simulink model "feedback_lin_RLS_soloR"  (R2023b)
settings: Solver=VariableStepAuto  StartTime=0.0  StopTime=10  RelTol=1e-3
undefined symbols (not defined in the file): A_ob, B_ob, C_ob, D_ob, k_aero, k_mag, k_mag_mod, Lc, Lc_mod, m, Rtot, Rtot_mod, theta, x1_eq0, x2_eq0, y0
libraries: simulink x6
settings Model: Creator=lollo  LastModifiedBy=lollo

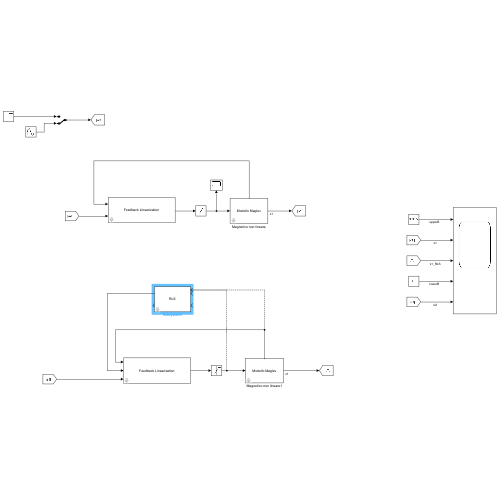
[thumbnail: Simulink's stored preview of the top-level diagram]
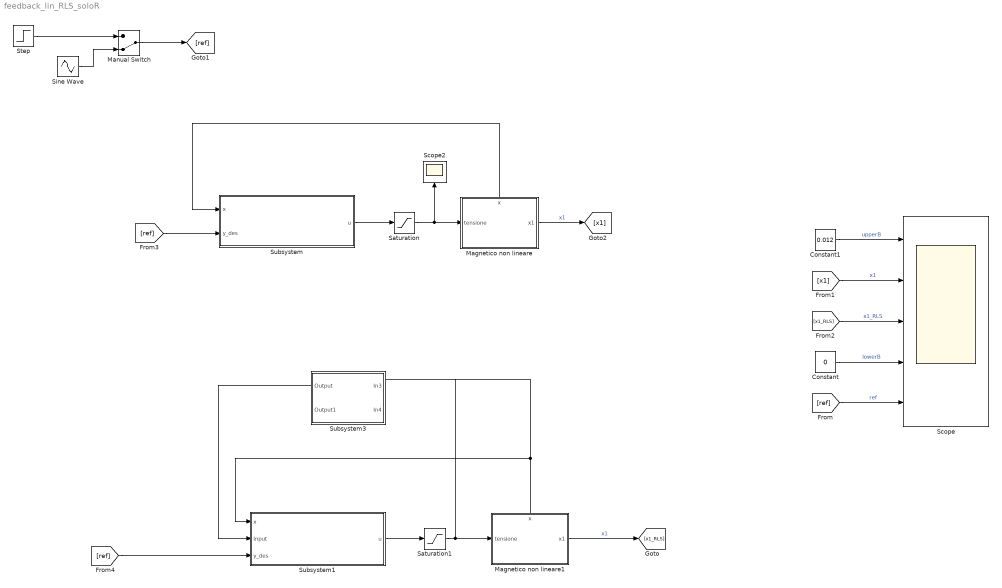
== system feedback_lin_RLS_soloR ==
  Constant : Constant  Value=0
  Constant1 : Constant  Value=0.012
  Magnetico non lineare : Subsystem  mask{dist=off, obs=on}
      mask prompts: dist "Aggiungere Disturbi"; obs "Observer invece di misura"
      settings: PortSchema="{\"entries\":[{\"content\":{\"sides\":[{\"content\":{\"connectorIds\":[\"In1\"]},\"type\":\"ConnectorPlacement.EquallySpacedRectSide\",\"uuid\":\"4c2628b7-19c4-4753-accd-078547eff280\"},{\"content\":{\"connectorIds\":[\"Out1\"],\"side\":\"RIGHT\"},\"type\":\"ConnectorPlacement.EquallySpacedRectSide\",\"uuid\":\"46f8a782-99b4-4db5-ac9e-879226864e1a\"},{\"content\":{\"connectorIds\":[\"Out2\"],\"side\":\"TOP\"},\"type\":\"ConnectorPlacement.EquallySpacedRectSide\",\"uuid\":\"e9ea6a3a-0b10-4f27-be26-5b91ce6de957\"}]},\"type\":\"ConnectorPlacement.EquallySpacedConnector\",\"uuid\":\"8380a659-82e1-48e4-be7e-4b84feeb9f50\"}],\"packageUris\":[\"http://schema.mathworks.com/mf0/Connector/R2020b\"],\"version\":\"1.0\"}"
      mask DialogControl DescGroupVar Prompt: MAGLEV
      mask DialogControl Maglev Prompt: Possibilità di aggiungere disturbi alla misura o di considerare gli observer (solo ridotto alla velocità). Inoltre possibilità di modificare i parametri del modello per testare robustezza
      mask DialogControl Disturbi Prompt: Disturbi
      mask Display: disp('Modello Maglev')
  Magnetico non lineare1 : Subsystem  mask{dist=on, obs=on}
      mask prompts: dist "Aggiungere Disturbi"; obs "Observer invece di misura"
      settings: PortSchema="{\"entries\":[{\"content\":{\"sides\":[{\"content\":{\"connectorIds\":[\"In1\"]},\"type\":\"ConnectorPlacement.EquallySpacedRectSide\",\"uuid\":\"4c2628b7-19c4-4753-accd-078547eff280\"},{\"content\":{\"connectorIds\":[\"Out1\"],\"side\":\"RIGHT\"},\"type\":\"ConnectorPlacement.EquallySpacedRectSide\",\"uuid\":\"46f8a782-99b4-4db5-ac9e-879226864e1a\"},{\"content\":{\"connectorIds\":[\"Out2\"],\"side\":\"TOP\"},\"type\":\"ConnectorPlacement.EquallySpacedRectSide\",\"uuid\":\"e9ea6a3a-0b10-4f27-be26-5b91ce6de957\"}]},\"type\":\"ConnectorPlacement.EquallySpacedConnector\",\"uuid\":\"8380a659-82e1-48e4-be7e-4b84feeb9f50\"}],\"packageUris\":[\"http://schema.mathworks.com/mf0/Connector/R2020b\"],\"version\":\"1.0\"}"
      mask DialogControl DescGroupVar Prompt: MAGLEV
      mask DialogControl Maglev Prompt: Possibilità di aggiungere disturbi alla misura o di considerare gli observer (solo ridotto alla velocità). Inoltre possibilità di modificare i parametri del modello per testare robustezza
      mask DialogControl Disturbi Prompt: Disturbi
      mask Display: disp('Modello Maglev')
  Manual Switch : ManualSwitch  CurrentSetting=0
  Saturation : Saturate  UpperLimit=23  LowerLimit=0
  Saturation1 : Saturate  UpperLimit=23  LowerLimit=0
  Scope : Scope  NumInputPorts=5
  Scope2 : Scope
  Sine Wave : Sin  Amplitude=0.001  Bias=0.003  Frequency=10  SampleTime=0
  Step : Step  Time=0  After=0.003  SampleTime=0
  Subsystem : Subsystem  mask{tau=0.003, p1=-100, p2=-60, p3=-70}
      mask DialogControl DescGroupVar Prompt: Feedback Linearization
      mask DialogControl DescTextVar Prompt: Tau corrisponde al tempo caratteristico del filtro per il calcolo delle derivate. k1, k2, k3 sono i poli della feedback linearization dei rispettivi stati
      mask Display: disp('Feedback Linearization')
  Subsystem1 : Subsystem  mask{tau=0.003, p1=-40, p2=-50, p3=-50}
      mask DialogControl DescGroupVar Prompt: Feedback Linearization
      mask DialogControl DescTextVar Prompt: Tau corrisponde al tempo caratteristico del filtro per il calcolo delle derivate. k1, k2, k3 sono i poli della feedback linearization dei rispettivi stati
      mask Display: disp('Feedback Linearization')
  Subsystem3 : Subsystem
      mask Display: disp('RLS')
  wires:
  Magnetico non lineare/2(x) -> Subsystem/1(x)
  Manual Switch/1 -> [ref]
  Subsystem/1(u) -> Saturation/1
  Saturation/1 -> Magnetico non lineare/1(tensione), Scope2/1
  Step/1 -> Manual Switch/1
  Sine Wave/1 -> Manual Switch/2
  Saturation1/1 -> Magnetico non lineare1/1(tensione)
  Magnetico non lineare1/2(x) -> Subsystem1/1(x)
  [ref] -> Subsystem1/3(y_des)
  Subsystem3/1(Output) -> Subsystem1/2(Input)
  Constant/1 -> Scope/4  "lowerB"
  [x1] -> Scope/2  "x1"
  [ref] -> Scope/5  "ref"
  Constant1/1 -> Scope/1  "upperB"
  Magnetico non lineare/1(x1) -> [x1]  "x1"
  [x1_RLS] -> Scope/3  "x1_RLS"
  Magnetico non lineare1/1(x1) -> [x1_RLS]  "x1"
  [ref] -> Subsystem/2(y_des)
  Subsystem1/1(u) -> Saturation1/1

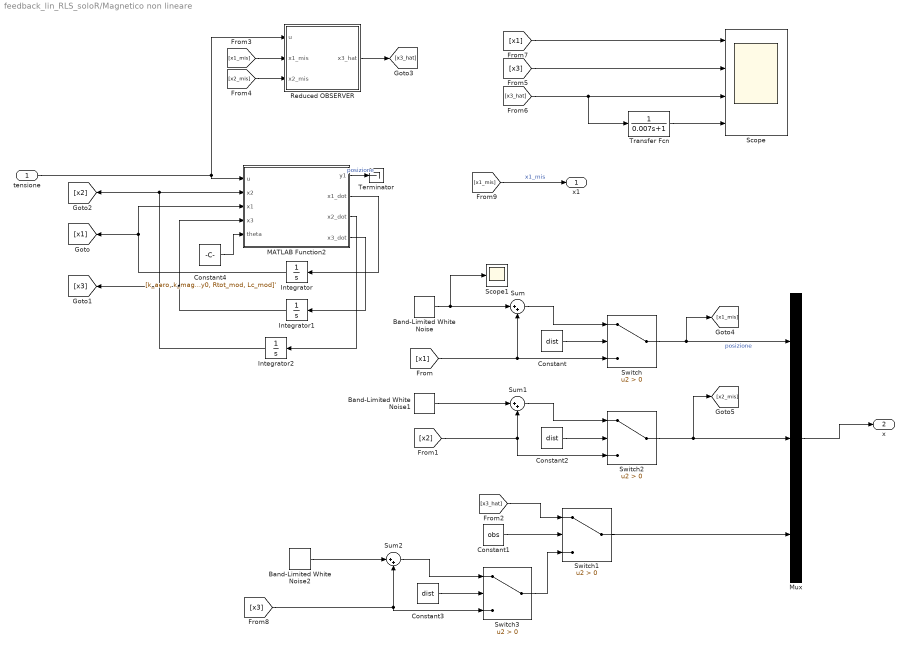
== system feedback_lin_RLS_soloR/Magnetico non lineare ==
  tensione : Inport
  Band-Limited White Noise : simulink/Sources/Band-Limited White Noise  Cov=[1e-10*0.002]  Ts=0.002  seed=[23341]
  Band-Limited White Noise1 : simulink/Sources/Band-Limited White Noise  Cov=[8.9934e-11*0.002]  Ts=0.002  seed=[23341]
  Band-Limited White Noise2 : simulink/Sources/Band-Limited White Noise  Cov=[8.9934e-11*0.002]  Ts=0.002  seed=[23341]
  Constant : Constant  Value=dist
  Constant1 : Constant  Value=obs
  Constant2 : Constant  Value=dist
  Constant3 : Constant  Value=dist
  Constant4 : Constant  Value=[k_aero, k_mag_mod, m, y0, Rtot_mod, Lc_mod]'
  Integrator : Integrator
  Integrator1 : Integrator
  Integrator2 : Integrator
  MATLAB Function2 : MATLAB Function  TreatAsAtomicUnit=on
  Mux : Mux  Inputs=3
  Reduced OBSERVER : Subsystem
  Scope : Scope  NumInputPorts=4
  Scope1 : Scope
  Sum : Sum  Inputs=|++
  Sum1 : Sum  Inputs=|++
  Sum2 : Sum  Inputs=|++
  Switch{,1..3} (4 alike) : Switch  Criteria=u2 > Threshold  SaturateOnIntegerOverflow=off  InputSameDT=off
  Terminator : Terminator
  Transfer Fcn : TransferFcn  Denominator=[0.007 1]
  x1 : Outport
  x : Outport  Port=2
  wires:
  tensione/1 -> Reduced OBSERVER/1(u), MATLAB Function2/1(u)
  Switch/1 -> [x1_mis], Mux/1  "posizione"
  MATLAB Function2/2(x1_dot) -> Integrator/1
  Integrator/1 -> MATLAB Function2/3(x1), [x1]
  MATLAB Function2/4(x3_dot) -> Integrator1/1
  Integrator1/1 -> [x3], MATLAB Function2/4(x3)
  [x1] -> Sum/2, Switch/3
  [x3_hat] -> Switch1/1
  Mux/1 -> x/1
  MATLAB Function2/3(x2_dot) -> Integrator2/1
  [x1_mis] -> Reduced OBSERVER/2(x1_mis)
  [x2_mis] -> Reduced OBSERVER/3(x2_mis)
  Reduced OBSERVER/1(x3_hat) -> [x3_hat]
  [x3_hat] -> Transfer Fcn/1, Scope/3
  [x3] -> Scope/2
  Integrator2/1 -> [x2], MATLAB Function2/2(x2)
  [x1] -> Scope/1
  Constant/1 -> Switch/2
  Band-Limited White Noise/1 -> Scope1/1, Sum/1
  Sum/1 -> Switch/1
  Constant1/1 -> Switch1/2
  Switch1/1 -> Mux/3
  Constant2/1 -> Switch2/2
  Switch2/1 -> [x2_mis], Mux/2
  Band-Limited White Noise1/1 -> Sum1/1
  Sum1/1 -> Switch2/1
  [x2] -> Sum1/2, Switch2/3
  Constant3/1 -> Switch3/2
  Switch3/1 -> Switch1/3
  Band-Limited White Noise2/1 -> Sum2/1
  Sum2/1 -> Switch3/1
  [x3] -> Sum2/2, Switch3/3
  Constant4/1 -> MATLAB Function2/5(theta)
  Transfer Fcn/1 -> Scope/4
  [x1_mis] -> x1/1  "x1_mis"
  MATLAB Function2/1(y1) -> Terminator/1  "posizione"

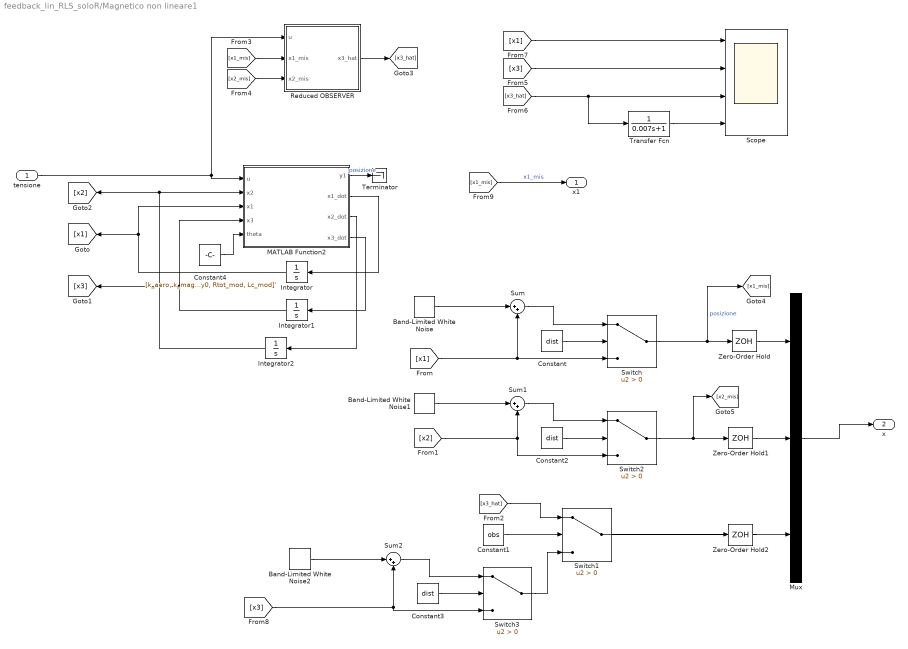
== system feedback_lin_RLS_soloR/Magnetico non lineare1 ==
  tensione : Inport
  Band-Limited White Noise : simulink/Sources/Band-Limited White Noise  Cov=[1e-8*0.002]  Ts=0.002  seed=[23341]
  Band-Limited White Noise1 : simulink/Sources/Band-Limited White Noise  Cov=[8.9934e-11*0.002]  Ts=0.002  seed=[23341]
  Band-Limited White Noise2 : simulink/Sources/Band-Limited White Noise  Cov=[8.9934e-11*0.002]  Ts=0.002  seed=[23341]
  Constant : Constant  Value=dist
  Constant1 : Constant  Value=obs
  Constant2 : Constant  Value=dist
  Constant3 : Constant  Value=dist
  Constant4 : Constant  Value=[k_aero, k_mag_mod, m, y0, Rtot_mod, Lc_mod]'
  Integrator : Integrator
  Integrator1 : Integrator
  Integrator2 : Integrator
  MATLAB Function2 : MATLAB Function  TreatAsAtomicUnit=on
  Mux : Mux  Inputs=3
  Reduced OBSERVER : Subsystem
  Scope : Scope  NumInputPorts=4
  Sum : Sum  Inputs=|++
  Sum1 : Sum  Inputs=|++
  Sum2 : Sum  Inputs=|++
  Switch{,1..3} (4 alike) : Switch  Criteria=u2 > Threshold  SaturateOnIntegerOverflow=off  InputSameDT=off
  Terminator : Terminator
  Transfer Fcn : TransferFcn  Denominator=[0.007 1]
  Zero-Order Hold : ZeroOrderHold  SampleTime=0.002
  Zero-Order Hold1 : ZeroOrderHold  SampleTime=0.002
  Zero-Order Hold2 : ZeroOrderHold  SampleTime=0.002
  x1 : Outport
  x : Outport  Port=2
  wires:
  tensione/1 -> Reduced OBSERVER/1(u), MATLAB Function2/1(u)
  Switch/1 -> [x1_mis], Zero-Order Hold/1  "posizione"
  MATLAB Function2/2(x1_dot) -> Integrator/1
  Integrator/1 -> MATLAB Function2/3(x1), [x1]
  MATLAB Function2/4(x3_dot) -> Integrator1/1
  Integrator1/1 -> [x3], MATLAB Function2/4(x3)
  [x1] -> Sum/2, Switch/3
  [x3_hat] -> Switch1/1
  Mux/1 -> x/1
  MATLAB Function2/3(x2_dot) -> Integrator2/1
  [x1_mis] -> Reduced OBSERVER/2(x1_mis)
  [x2_mis] -> Reduced OBSERVER/3(x2_mis)
  Reduced OBSERVER/1(x3_hat) -> [x3_hat]
  [x3_hat] -> Transfer Fcn/1, Scope/3
  [x3] -> Scope/2
  Integrator2/1 -> [x2], MATLAB Function2/2(x2)
  [x1] -> Scope/1
  Constant/1 -> Switch/2
  Band-Limited White Noise/1 -> Sum/1
  Sum/1 -> Switch/1
  Constant1/1 -> Switch1/2
  Switch1/1 -> Zero-Order Hold2/1
  Constant2/1 -> Switch2/2
  Switch2/1 -> [x2_mis], Zero-Order Hold1/1
  Band-Limited White Noise1/1 -> Sum1/1
  Sum1/1 -> Switch2/1
  [x2] -> Sum1/2, Switch2/3
  Constant3/1 -> Switch3/2
  Switch3/1 -> Switch1/3
  Band-Limited White Noise2/1 -> Sum2/1
  Sum2/1 -> Switch3/1
  [x3] -> Sum2/2, Switch3/3
  Constant4/1 -> MATLAB Function2/5(theta)
  Transfer Fcn/1 -> Scope/4
  [x1_mis] -> x1/1  "x1_mis"
  MATLAB Function2/1(y1) -> Terminator/1  "posizione"
  Zero-Order Hold/1 -> Mux/1
  Zero-Order Hold1/1 -> Mux/2
  Zero-Order Hold2/1 -> Mux/3

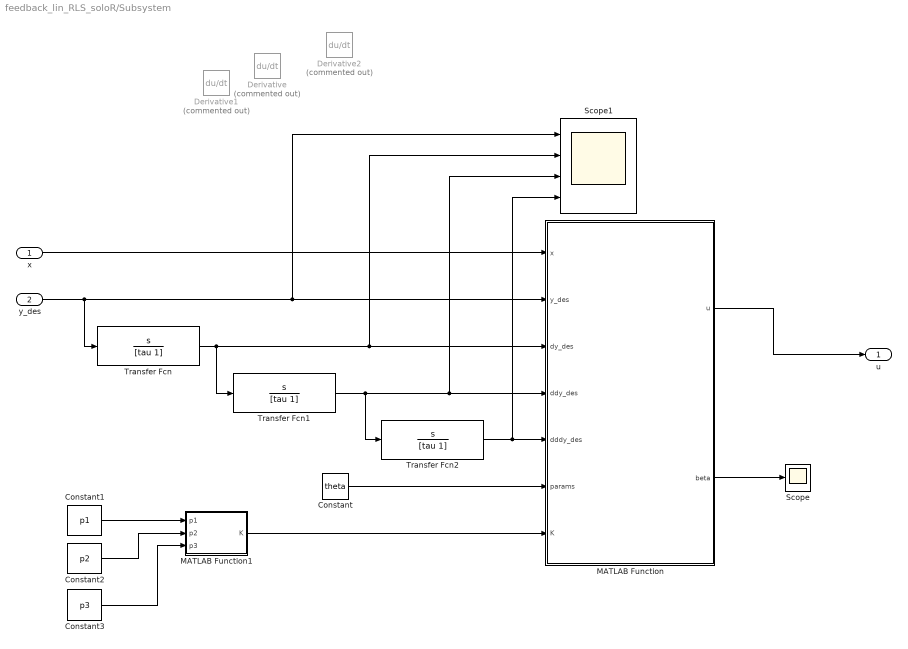
== system feedback_lin_RLS_soloR/Subsystem ==
  x : Inport
  y_des : Inport  Port=2
  Constant : Constant  Value=theta
  Constant1 : Constant  Value=p1
  Constant2 : Constant  Value=p2
  Constant3 : Constant  Value=p3
  Derivative : Derivative  Commented=on
  Derivative1 : Derivative  Commented=on
  Derivative2 : Derivative  Commented=on
  MATLAB Function : MATLAB Function  TreatAsAtomicUnit=on
  MATLAB Function1 : MATLAB Function  TreatAsAtomicUnit=on
  Scope : Scope
  Scope1 : Scope  NumInputPorts=4
  Transfer Fcn : TransferFcn  Numerator=[1 0]  Denominator=[tau 1]
  Transfer Fcn1 : TransferFcn  Numerator=[1 0]  Denominator=[tau 1]
  Transfer Fcn2 : TransferFcn  Numerator=[1 0]  Denominator=[tau 1]
  u : Outport
  wires:
  y_des/1 -> Transfer Fcn/1, MATLAB Function/2(y_des), Scope1/1
  x/1 -> MATLAB Function/1(x)
  MATLAB Function/1(u) -> u/1
  Transfer Fcn/1 -> MATLAB Function/3(dy_des), Scope1/2, Transfer Fcn1/1
  Constant/1 -> MATLAB Function/6(params)
  Transfer Fcn1/1 -> Transfer Fcn2/1, Scope1/3, MATLAB Function/4(ddy_des)
  MATLAB Function/2(beta) -> Scope/1
  Transfer Fcn2/1 -> Scope1/4, MATLAB Function/5(dddy_des)
  MATLAB Function1/1(K) -> MATLAB Function/7(K)
  Constant3/1 -> MATLAB Function1/3(p3)
  Constant2/1 -> MATLAB Function1/2(p2)
  Constant1/1 -> MATLAB Function1/1(p1)

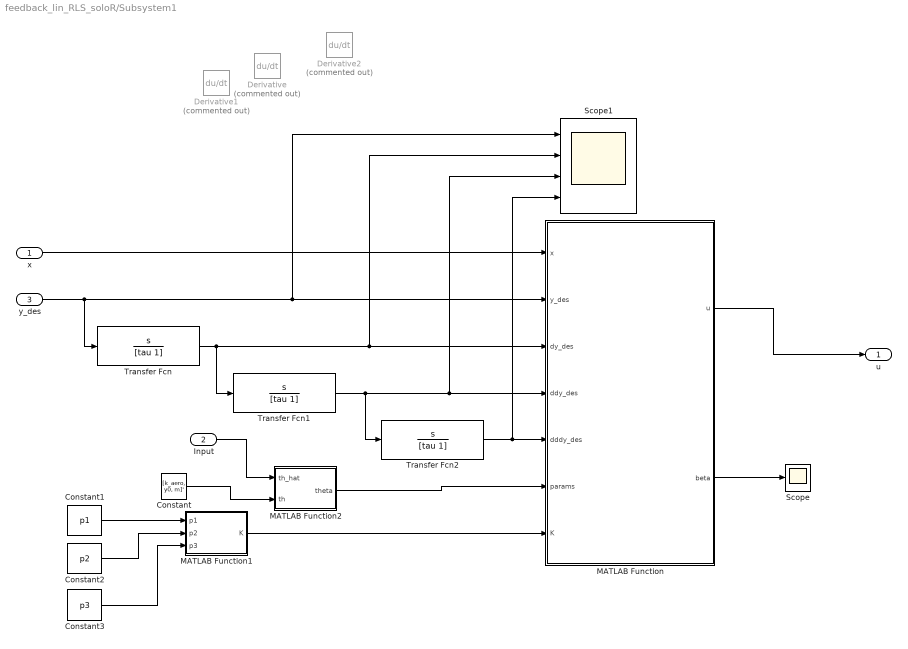
== system feedback_lin_RLS_soloR/Subsystem1 ==
  x : Inport
  Input : Inport  Port=2
  y_des : Inport  Port=3
  Constant : Constant  Value=[k_aero, y0, m]'
  Constant1 : Constant  Value=p1
  Constant2 : Constant  Value=p2
  Constant3 : Constant  Value=p3
  Derivative : Derivative  Commented=on
  Derivative1 : Derivative  Commented=on
  Derivative2 : Derivative  Commented=on
  MATLAB Function : MATLAB Function  TreatAsAtomicUnit=on
  MATLAB Function1 : MATLAB Function  TreatAsAtomicUnit=on
  MATLAB Function2 : MATLAB Function  TreatAsAtomicUnit=on
  Scope : Scope
  Scope1 : Scope  NumInputPorts=4
  Transfer Fcn : TransferFcn  Numerator=[1 0]  Denominator=[tau 1]
  Transfer Fcn1 : TransferFcn  Numerator=[1 0]  Denominator=[tau 1]
  Transfer Fcn2 : TransferFcn  Numerator=[1 0]  Denominator=[tau 1]
  u : Outport
  wires:
  y_des/1 -> Transfer Fcn/1, MATLAB Function/2(y_des), Scope1/1
  x/1 -> MATLAB Function/1(x)
  MATLAB Function/1(u) -> u/1
  Transfer Fcn/1 -> MATLAB Function/3(dy_des), Scope1/2, Transfer Fcn1/1
  MATLAB Function2/1(theta) -> MATLAB Function/6(params)
  Transfer Fcn1/1 -> Transfer Fcn2/1, Scope1/3, MATLAB Function/4(ddy_des)
  MATLAB Function/2(beta) -> Scope/1
  Transfer Fcn2/1 -> Scope1/4, MATLAB Function/5(dddy_des)
  MATLAB Function1/1(K) -> MATLAB Function/7(K)
  Constant3/1 -> MATLAB Function1/3(p3)
  Constant2/1 -> MATLAB Function1/2(p2)
  Constant1/1 -> MATLAB Function1/1(p1)
  Input/1 -> MATLAB Function2/1(th_hat)
  Constant/1 -> MATLAB Function2/2(th)

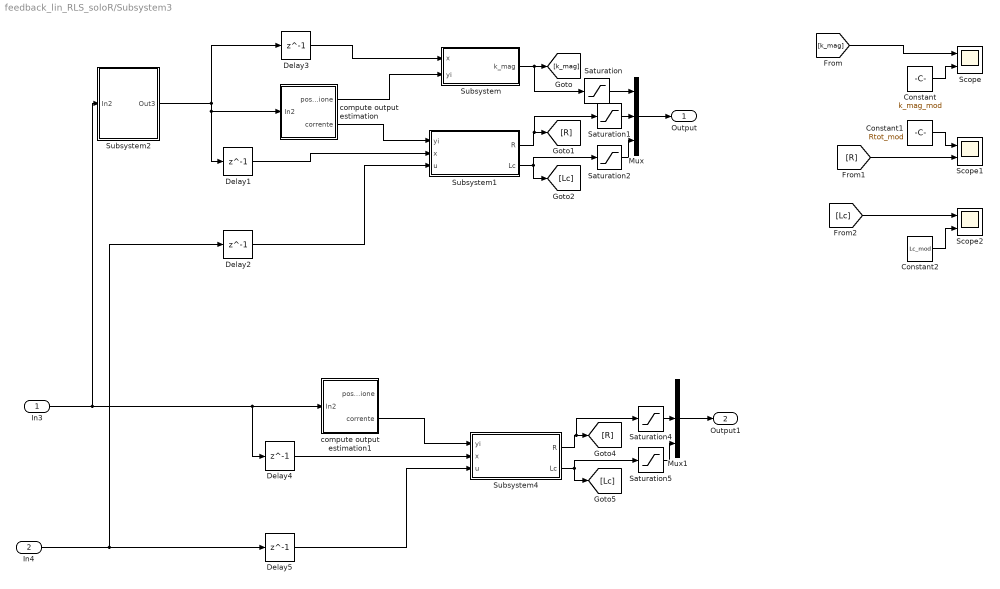
== system feedback_lin_RLS_soloR/Subsystem3 ==
  In3 : Inport
  In4 : Inport  Port=2
  Constant : Constant  Value=k_mag_mod
  Constant1 : Constant  Value=Rtot_mod
  Constant2 : Constant  Value=Lc_mod
  Delay{1..2,4..5} (4 alike) : Delay  DelayLength=1  InitialCondition=0
  Delay3 : Delay  DelayLength=1  InitialCondition=[0, 0, 0]'
  Mux : Mux  Inputs=3
  Mux1 : Mux  Inputs=3
  Saturation : Saturate  UpperLimit=1e-4  LowerLimit=1e-6
  Saturation1 : Saturate  UpperLimit=20  LowerLimit=0
  Saturation2 : Saturate  UpperLimit=2  LowerLimit=0
  Saturation4 : Saturate  UpperLimit=20  LowerLimit=0
  Saturation5 : Saturate  UpperLimit=2  LowerLimit=0
  Scope : Scope  NumInputPorts=2
  Scope1 : Scope  NumInputPorts=2
  Scope2 : Scope  NumInputPorts=2
  Subsystem : Subsystem  mask{th0=k_mag, S0=eye(1)/100, mu=0.98}
      mask prompts: th0 "Theta init"; mu "Forgetting factor"
      mask Display: disp('RLS (k_mag)')
  Subsystem1 : Subsystem  mask{th0=[Rtot; Lc], S0=eye(2)/10, mu=0.99}
      mask prompts: th0 "Theta init"; mu "Forgetting Factor"
      mask Display: disp('RLS (R, Lc)')
  Subsystem2 : Subsystem
  Subsystem4 : Subsystem  mask{th0=[Rtot; Lc], S0=eye(2)/10, mu=0.99}
      mask prompts: th0 "Theta init"; mu "Forgetting Factor"
      mask Display: disp('RLS (R, Lc)')
  compute output estimation : Subsystem
  compute output estimation1 : Subsystem
  Output : Outport
  Output1 : Outport  Port=2
  wires:
  Delay2/1 -> Subsystem1/3(u)
  Delay3/1 -> Subsystem/1(x)
  compute output estimation/1(posizione) -> Subsystem/2(yi)
  compute output estimation/2(corrente) -> Subsystem1/1(yi)
  Delay1/1 -> Subsystem1/2(x)
  Constant/1 -> Scope/2
  Constant1/1 -> Scope1/1
  Constant2/1 -> Scope2/2
  Subsystem/1(k_mag) -> Saturation/1, [k_mag]
  Subsystem1/1(R) -> Saturation1/1, [R]
  Subsystem1/2(Lc) -> [Lc], Saturation2/1
  [k_mag] -> Scope/1
  [R] -> Scope1/2
  [Lc] -> Scope2/1
  Mux/1 -> Output/1
  Subsystem2/1(Out3) -> Delay1/1, compute output estimation/1(In2), Delay3/1
  Saturation/1 -> Mux/1
  Saturation1/1 -> Mux/2
  Saturation2/1 -> Mux/3
  Saturation5/1 -> Mux1/3
  In3/1 -> Delay4/1, compute output estimation1/1(In2), Subsystem2/1(In2)
  Saturation4/1 -> Mux1/2
  Subsystem4/1(R) -> Saturation4/1, [R]
  Delay4/1 -> Subsystem4/2(x)
  Mux1/1 -> Output1/1
  compute output estimation1/2(corrente) -> Subsystem4/1(yi)
  Subsystem4/2(Lc) -> [Lc], Saturation5/1
  Delay5/1 -> Subsystem4/3(u)
  In4/1 -> Delay2/1, Delay5/1

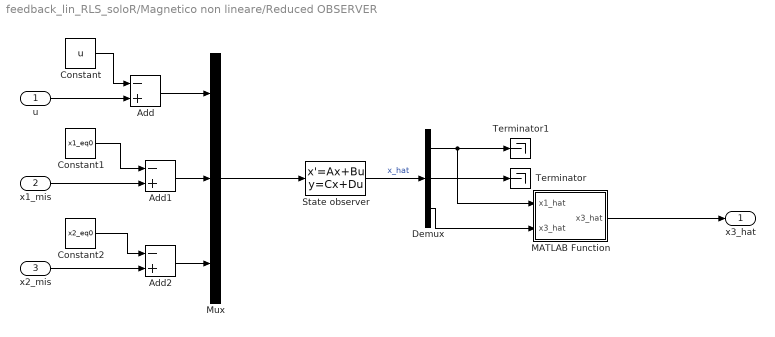
== system feedback_lin_RLS_soloR/Magnetico non lineare/Reduced OBSERVER ==
  u : Inport
  x1_mis : Inport  Port=2
  x2_mis : Inport  Port=3
  Add : Sum  Inputs=-+
  Add1 : Sum  Inputs=-+
  Add2 : Sum  Inputs=-+
  Constant : Constant  Value=u
  Constant1 : Constant  Value=x1_eq0
  Constant2 : Constant  Value=x2_eq0
  Demux : Demux  Outputs=3
  MATLAB Function : MATLAB Function  TreatAsAtomicUnit=on
  Mux : Mux  Inputs=3
  State observer : StateSpace  A=A_ob  B=B_ob  C=C_ob  D=D_ob  InitialCondition=[0;0;0]  ParameterTunability=Unconstrained
  Terminator : Terminator
  Terminator1 : Terminator
  x3_hat : Outport
  wires:
  x1_mis/1 -> Add1/2
  u/1 -> Add/2
  Mux/1 -> State observer/1
  State observer/1 -> Demux/1  "x_hat"
  Demux/1 -> MATLAB Function/1(x1_hat), Terminator1/1
  Demux/2 -> Terminator/1
  Constant/1 -> Add/1
  Constant1/1 -> Add1/1
  Constant2/1 -> Add2/1
  x2_mis/1 -> Add2/2
  Add/1 -> Mux/1
  Add1/1 -> Mux/2
  Add2/1 -> Mux/3
  MATLAB Function/1(x3_hat) -> x3_hat/1
  Demux/3 -> MATLAB Function/2("x3_hat ")

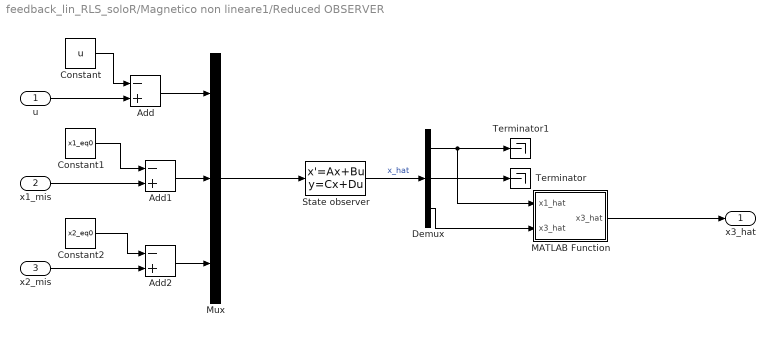
== system feedback_lin_RLS_soloR/Magnetico non lineare1/Reduced OBSERVER ==
  u : Inport
  x1_mis : Inport  Port=2
  x2_mis : Inport  Port=3
  Add : Sum  Inputs=-+
  Add1 : Sum  Inputs=-+
  Add2 : Sum  Inputs=-+
  Constant : Constant  Value=u
  Constant1 : Constant  Value=x1_eq0
  Constant2 : Constant  Value=x2_eq0
  Demux : Demux  Outputs=3
  MATLAB Function : MATLAB Function  TreatAsAtomicUnit=on
  Mux : Mux  Inputs=3
  State observer : StateSpace  A=A_ob  B=B_ob  C=C_ob  D=D_ob  InitialCondition=[0;0;0]  ParameterTunability=Unconstrained
  Terminator : Terminator
  Terminator1 : Terminator
  x3_hat : Outport
  wires:
  x1_mis/1 -> Add1/2
  u/1 -> Add/2
  Mux/1 -> State observer/1
  State observer/1 -> Demux/1  "x_hat"
  Demux/1 -> MATLAB Function/1(x1_hat), Terminator1/1
  Demux/2 -> Terminator/1
  Constant/1 -> Add/1
  Constant1/1 -> Add1/1
  Constant2/1 -> Add2/1
  x2_mis/1 -> Add2/2
  Add/1 -> Mux/1
  Add1/1 -> Mux/2
  Add2/1 -> Mux/3
  MATLAB Function/1(x3_hat) -> x3_hat/1
  Demux/3 -> MATLAB Function/2("x3_hat ")

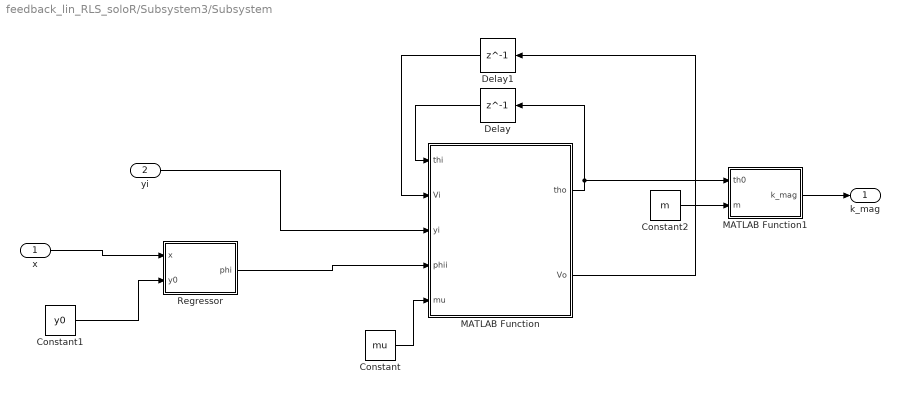
== system feedback_lin_RLS_soloR/Subsystem3/Subsystem ==
  x : Inport
  yi : Inport  Port=2
  Constant : Constant  Value=mu
  Constant1 : Constant  Value=y0
  Constant2 : Constant  Value=m
  Delay : Delay  DelayLength=1  InitialCondition=th0*0.002^2/m
  Delay1 : Delay  DelayLength=1  InitialCondition=inv(S0)
  MATLAB Function : MATLAB Function  TreatAsAtomicUnit=on
  MATLAB Function1 : MATLAB Function  TreatAsAtomicUnit=on
  Regressor : MATLAB Function  TreatAsAtomicUnit=on
  k_mag : Outport
  wires:
  yi/1 -> MATLAB Function/3(yi)
  Constant/1 -> MATLAB Function/5(mu)
  Delay/1 -> MATLAB Function/1(thi)
  Delay1/1 -> MATLAB Function/2(Vi)
  MATLAB Function/1(tho) -> MATLAB Function1/1(th0), Delay/1
  Regressor/1(phi) -> MATLAB Function/4(phii)
  MATLAB Function/2(Vo) -> Delay1/1
  x/1 -> Regressor/1(x)
  Constant1/1 -> Regressor/2(y0)
  MATLAB Function1/1(k_mag) -> k_mag/1
  Constant2/1 -> MATLAB Function1/2(m)

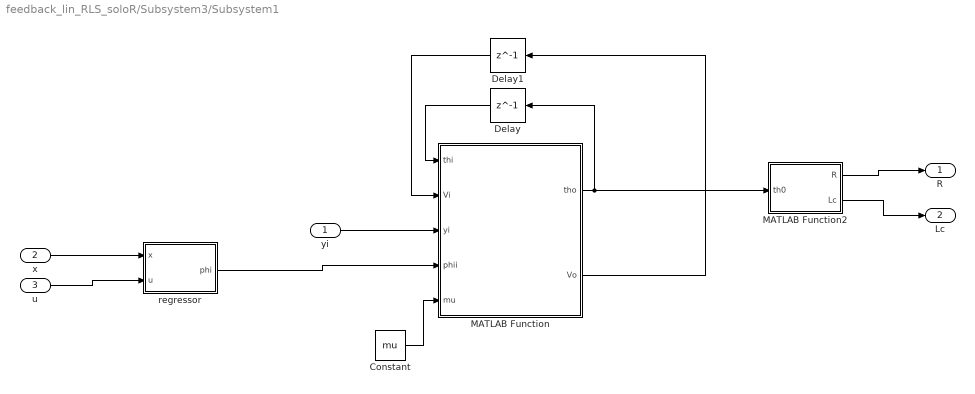
== system feedback_lin_RLS_soloR/Subsystem3/Subsystem1 ==
  yi : Inport
  x : Inport  Port=2
  u : Inport  Port=3
  Constant : Constant  Value=mu
  Delay : Delay  DelayLength=1  InitialCondition=[th0(1)*0.002/th0(2); 0.002/th0(2)]
  Delay1 : Delay  DelayLength=1  InitialCondition=inv(S0)
  MATLAB Function : MATLAB Function  TreatAsAtomicUnit=on
  MATLAB Function2 : MATLAB Function  TreatAsAtomicUnit=on
  regressor : MATLAB Function  TreatAsAtomicUnit=on
  R : Outport
  Lc : Outport  Port=2
  wires:
  yi/1 -> MATLAB Function/3(yi)
  Constant/1 -> MATLAB Function/5(mu)
  Delay/1 -> MATLAB Function/1(thi)
  Delay1/1 -> MATLAB Function/2(Vi)
  MATLAB Function/1(tho) -> MATLAB Function2/1(th0), Delay/1
  regressor/1(phi) -> MATLAB Function/4(phii)
  MATLAB Function/2(Vo) -> Delay1/1
  x/1 -> regressor/1(x)
  u/1 -> regressor/2(u)
  MATLAB Function2/1(R) -> R/1
  MATLAB Function2/2(Lc) -> Lc/1

== system feedback_lin_RLS_soloR/Subsystem3/Subsystem2 ==
  In2 : Inport
  Demux : Demux  Outputs=3
  Mux1 : Mux  Inputs=3
  Out3 : Outport
  wires:
  Mux1/1 -> Out3/1
  In2/1 -> Demux/1
  Demux/3 -> Mux1/3
  Demux/2 -> Mux1/2
  Demux/1 -> Mux1/1

== system feedback_lin_RLS_soloR/Subsystem3/Subsystem4 ==
  yi : Inport
  x : Inport  Port=2
  u : Inport  Port=3
  Constant : Constant  Value=mu
  Delay : Delay  DelayLength=1  InitialCondition=[th0(1)*0.002/th0(2); 0.002/th0(2)]
  Delay1 : Delay  DelayLength=1  InitialCondition=inv(S0)
  MATLAB Function : MATLAB Function  TreatAsAtomicUnit=on
  MATLAB Function2 : MATLAB Function  TreatAsAtomicUnit=on
  regressor : MATLAB Function  TreatAsAtomicUnit=on
  R : Outport
  Lc : Outport  Port=2
  wires:
  yi/1 -> MATLAB Function/3(yi)
  Constant/1 -> MATLAB Function/5(mu)
  Delay/1 -> MATLAB Function/1(thi)
  Delay1/1 -> MATLAB Function/2(Vi)
  MATLAB Function/1(tho) -> MATLAB Function2/1(th0), Delay/1
  regressor/1(phi) -> MATLAB Function/4(phii)
  MATLAB Function/2(Vo) -> Delay1/1
  x/1 -> regressor/1(x)
  u/1 -> regressor/2(u)
  MATLAB Function2/1(R) -> R/1
  MATLAB Function2/2(Lc) -> Lc/1

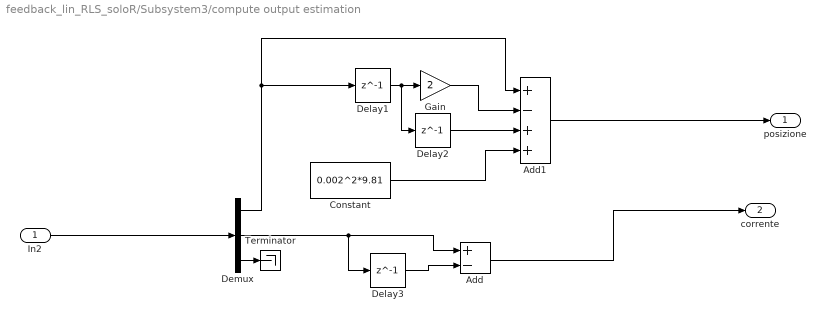
== system feedback_lin_RLS_soloR/Subsystem3/compute output estimation ==
  In2 : Inport
  Add : Sum  Inputs=+-
  Add1 : Sum  Inputs=+-++
  Constant : Constant  Value=0.002^2*9.81
  Delay1 : Delay  DelayLength=1
  Delay2 : Delay  DelayLength=1
  Delay3 : Delay  DelayLength=1
  Demux : Demux  Outputs=3
  Gain : Gain  Gain=2
  Terminator : Terminator
  posizione : Outport
  corrente : Outport  Port=2
  wires:
  In2/1 -> Demux/1
  Demux/3 -> Terminator/1
  Demux/2 -> Delay3/1, Add/1
  Delay3/1 -> Add/2
  Add/1 -> corrente/1
  Demux/1 -> Delay1/1, Add1/1
  Delay1/1 -> Delay2/1, Gain/1
  Gain/1 -> Add1/2
  Delay2/1 -> Add1/3
  Constant/1 -> Add1/4
  Add1/1 -> posizione/1

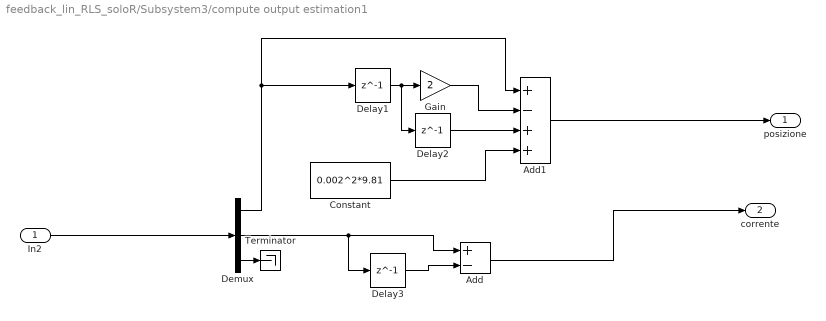
== system feedback_lin_RLS_soloR/Subsystem3/compute output estimation1 ==
  In2 : Inport
  Add : Sum  Inputs=+-
  Add1 : Sum  Inputs=+-++
  Constant : Constant  Value=0.002^2*9.81
  Delay1 : Delay  DelayLength=1
  Delay2 : Delay  DelayLength=1
  Delay3 : Delay  DelayLength=1
  Demux : Demux  Outputs=3
  Gain : Gain  Gain=2
  Terminator : Terminator
  posizione : Outport
  corrente : Outport  Port=2
  wires:
  In2/1 -> Demux/1
  Demux/3 -> Terminator/1
  Demux/2 -> Delay3/1, Add/1
  Delay3/1 -> Add/2
  Add/1 -> corrente/1
  Demux/1 -> Delay1/1, Add1/1
  Delay1/1 -> Delay2/1, Gain/1
  Gain/1 -> Add1/2
  Delay2/1 -> Add1/3
  Constant/1 -> Add1/4
  Add1/1 -> posizione/1

== matlab function feedback_lin_RLS_soloR/Subsystem3/Subsystem1/MATLAB Function2 ==
  data: th0 input; R output; Lc output
function [R, Lc] = fcn(th0)

    R = th0(1)/th0(2);
    Lc = 0.002/th0(2);



end

== matlab function feedback_lin_RLS_soloR/Subsystem3/Subsystem/MATLAB Function1 ==
  data: th0 input; k_mag output; m input
function k_mag = fcn(th0, m)

    k_mag = th0*m/0.002^2;



end

== matlab function feedback_lin_RLS_soloR/Magnetico non lineare1/MATLAB Function2 ==
  data: u input; y1 output; x2 input; x1_dot output; x2_dot output; x1 input; x3 input; x3_dot output; theta input
function [y1,x1_dot, x2_dot, x3_dot] = fcn(u, x2, x1, x3, theta)
    k_aero = theta(1, 1);
    k_mag = theta(2, 1);
    m = theta(3, 1);
    y0 = theta(4, 1);
    Rtot = theta(5, 1);
    Lc = theta(6, 1);
    g = 9.81;
    
    x2_dot = 1/Lc*(-Rtot*x2 + u);

    x1_dot = x3;
    if x1 < y0
        x3_dot = (k_mag/m)*(x2/(y0-x1))^2 - g;
    else
        x1 = 0.012;
        x3_dot = 0;
        x3 = 0;
    end

    
    % condizioni
    if x1 <=0 && x3_dot < 0
        x1 = 0;
        x3 = 0;
        x3_dot = 0;
    end
y1 = x1;

== matlab function feedback_lin_RLS_soloR/Magnetico non lineare1/Reduced OBSERVER/MATLAB Function ==
  data: x1_hat input; x3_hat output; x3_hat input
function x3_hat = fcn(x1_hat, x3_hat)

    if x1_hat<=0 && x3_hat<=0
        x3_hat=0;
    end
end

== matlab function feedback_lin_RLS_soloR/Subsystem1/MATLAB Function ==
  data: x input; u output; y_des input; dy_des input; ddy_des input; dddy_des input; params input; K input; beta output
function [u, beta] = feedback_linearization_control(x, y_des, dy_des, ddy_des, dddy_des, params, K)
    % Estrai parametri
    k_aero = params(1);
    k_mag  = params(2);
    m      = params(3);
    y0     = params(4);
    Rtot   = params(5);
    Lc     = params(6);
    g      = 9.81;

    % Stati
    x1 = x(1); % posizione
    x2 = x(2); % corrente
    x3 = x(3); % velocità

    % Derivate
    denom = (y0 - x1);
    if denom <= 0
        warning('Denominatore nullo o negativo: instabilità elettromagnetica');
    end

    % Accelerazione reale
    xdot3 = (k_aero/m)*x3 + (k_mag/m)*(x2 / denom)^2 - g;

    % Derivate parziali
    dBdx1 = (2 * k_mag * x2^2) / (m * denom^3);
    dBdx2 = (2 * k_mag * x2)   / (m * denom^2);
    dBdx3 = (k_aero/m);

    % Corrente senza ingresso (per calcolo alpha)
    dx2_nou = -(Rtot/Lc)*x2;

    % Parte non lineare (α) e lineare (β)
    alpha = dBdx1 * x3 + dBdx2 * dx2_nou + dBdx3 * xdot3;
    beta  = dBdx2 * (1/Lc);

    if abs(beta) < 1e-6
        warning('Beta troppo piccolo: possibile instabilità numerica');
        u = 5;
        return;
    end

    % Errore e controllore
    e   = x1 - y_des;
    de  = x3 - dy_des;
    ae  = xdot3 - ddy_des;

    

    % Guadagni
    k1 = K(1);
    k2 = K(2);
    k3 = K(3);
    

    % Ingresso virtuale
    % v = p(1, 1)*dddy_des + p(1, 2)*e + p(1, 3)*de + p(1, 4)*ae;
    v = dddy_des - k1*e - k2*de - k3*ae;
    % v = -k1*x1 - k2*x2 - k3*x3;

    % Controllo reale
    u = (v - alpha) / beta;
end

== matlab function feedback_lin_RLS_soloR/Subsystem1/MATLAB Function1 ==
  data: p1 input; K output; p2 input; p3 input
function K = fcn(p1, p2, p3)

    desired_roots = [p1, p2, p3];
    coeff = poly(desired_roots);     % s^3 + a2*s^2 + a1*s + a0
    K = fliplr(coeff(2:end));

== matlab function feedback_lin_RLS_soloR/Subsystem1/MATLAB Function2 ==
  data: th_hat input; theta output; th input
function theta = fcn(th_hat, th)

    k_mag = th_hat(1);
    Rtot = th_hat(2);
    Lc = th_hat(3);
    k_aero = th(1);
    y0 = th(2);
    m = th(3);

    theta = [k_aero, k_mag, m, y0, Rtot, Lc]';


end

== matlab function feedback_lin_RLS_soloR/Subsystem3/Subsystem4/MATLAB Function ==
  data: thi input; tho output; Vi input; yi input; phii input; Vo output; mu input
function [tho,Vo] = updaterule(thi,Vi,yi,phii,mu)

Vo = Vi/mu - (Vi*phii*phii'*Vi)/(mu+phii'*Vi*phii)/mu;
tho = thi + Vo*phii*(yi-phii'*thi);

== matlab function feedback_lin_RLS_soloR/Magnetico non lineare/Reduced OBSERVER/MATLAB Function ==
  data: x1_hat input; x3_hat output; x3_hat input
function x3_hat = fcn(x1_hat, x3_hat)

    if x1_hat<=0 && x3_hat<=0
        x3_hat=0;
    end
end

== matlab function feedback_lin_RLS_soloR/Subsystem3/Subsystem4/MATLAB Function2 ==
  data: th0 input; R output; Lc output
function [R, Lc] = fcn(th0)

    R = th0(1)/th0(2);
    Lc = 0.002/th0(2);



end

== matlab function feedback_lin_RLS_soloR/Subsystem3/Subsystem4/regressor ==
  data: x input; u input; phi output
function phi = fcn(x, u)

    phi = [-x(2); u];

end

== matlab function feedback_lin_RLS_soloR/Subsystem/MATLAB Function ==
  data: x input; u output; y_des input; dy_des input; ddy_des input; dddy_des input; params input; K input; beta output
function [u, beta] = feedback_linearization_control(x, y_des, dy_des, ddy_des, dddy_des, params, K)
    % Estrai parametri
    k_aero = params(1);
    k_mag  = params(2);
    m      = params(3);
    y0     = params(4);
    Rtot   = params(5);
    Lc     = params(6);
    g      = 9.81;

    % Stati
    x1 = x(1); % posizione
    x2 = x(2); % corrente
    x3 = x(3); % velocità

    % Derivate
    denom = (y0 - x1);
    if denom <= 0
        warning('Denominatore nullo o negativo: instabilità elettromagnetica');
    end

    % Accelerazione reale
    xdot3 = (k_aero/m)*x3 + (k_mag/m)*(x2 / denom)^2 - g;

    % Derivate parziali
    dBdx1 = (2 * k_mag * x2^2) / (m * denom^3);
    dBdx2 = (2 * k_mag * x2)   / (m * denom^2);
    dBdx3 = (k_aero/m);

    % Corrente senza ingresso (per calcolo alpha)
    dx2_nou = -(Rtot/Lc)*x2;

    % Parte non lineare (α) e lineare (β)
    alpha = dBdx1 * x3 + dBdx2 * dx2_nou + dBdx3 * xdot3;
    beta  = dBdx2 * (1/Lc);

    if abs(beta) < 1e-6
        warning('Beta troppo piccolo: possibile instabilità numerica');
        u = 5;
        return;
    end

    % Errore e controllore
    e   = x1 - y_des;
    de  = x3 - dy_des;
    ae  = xdot3 - ddy_des;

    

    % Guadagni
    k1 = K(1);
    k2 = K(2);
    k3 = K(3);
    

    % Ingresso virtuale
    % v = p(1, 1)*dddy_des + p(1, 2)*e + p(1, 3)*de + p(1, 4)*ae;
    v = dddy_des - k1*e - k2*de - k3*ae;
    % v = -k1*x1 - k2*x2 - k3*x3;

    % Controllo reale
    u = (v - alpha) / beta;
end

== matlab function feedback_lin_RLS_soloR/Subsystem/MATLAB Function1 ==
  data: p1 input; K output; p2 input; p3 input
function K = fcn(p1, p2, p3)

    desired_roots = [p1, p2, p3];
    coeff = poly(desired_roots);     % s^3 + a2*s^2 + a1*s + a0
    K = fliplr(coeff(2:end));

== matlab function feedback_lin_RLS_soloR/Magnetico non lineare/MATLAB Function2 ==
  data: u input; y1 output; x2 input; x1_dot output; x2_dot output; x1 input; x3 input; x3_dot output; theta input
function [y1,x1_dot, x2_dot, x3_dot] = fcn(u, x2, x1, x3, theta)
    k_aero = theta(1, 1);
    k_mag = theta(2, 1);
    m = theta(3, 1);
    y0 = theta(4, 1);
    Rtot = theta(5, 1);
    Lc = theta(6, 1);
    g = 9.81;
    
    x2_dot = 1/Lc*(-Rtot*x2 + u);

    x1_dot = x3;
    if x1 < y0
        x3_dot = (k_mag/m)*(x2/(y0-x1))^2 - g;
    else
        x1 = 0.012;
        x3_dot = 0;
        x3 = 0;
    end

    
    % condizioni
    if x1 <=0 && x3_dot < 0
        x1 = 0;
        x3 = 0;
        x3_dot = 0;
    end
y1 = x1;

== matlab function feedback_lin_RLS_soloR/Subsystem3/Subsystem/MATLAB Function ==
  data: thi input; tho output; Vi input; yi input; phii input; Vo output; mu input
function [tho,Vo] = updaterule(thi,Vi,yi,phii,mu)

Vo = Vi/mu - (Vi*phii*phii'*Vi)/(mu+phii'*Vi*phii)/mu;
tho = thi + Vo*phii*(yi-phii'*thi);

== matlab function feedback_lin_RLS_soloR/Subsystem3/Subsystem/Regressor ==
  data: x input; phi output; y0 input
function phi = fcn(x, y0)
    
    phi = (x(2)/(y0 - x(1)))^2;
    
end

== matlab function feedback_lin_RLS_soloR/Subsystem3/Subsystem1/MATLAB Function ==
  data: thi input; tho output; Vi input; yi input; phii input; Vo output; mu input
function [tho,Vo] = updaterule(thi,Vi,yi,phii,mu)

Vo = Vi/mu - (Vi*phii*phii'*Vi)/(mu+phii'*Vi*phii)/mu;
tho = thi + Vo*phii*(yi-phii'*thi);

== matlab function feedback_lin_RLS_soloR/Subsystem3/Subsystem1/regressor ==
  data: x input; u input; phi output
function phi = fcn(x, u)

    phi = [-x(2); u];

end
